simulink model "trialmk"  (R2017b)
settings: Solver=VariableStepAuto  StartTime=0.0  StopTime=10.0  RelTol=1e-3
values from neighbouring files (symbols this model uses):
  traj_freq = 1001    [basic_3link_plantraj3_emptry.m]
undefined symbols (not defined in the file or in its folder): FDab, planar
libraries: simulink x4
settings Model: Creator=USER  LastModifiedBy=USER

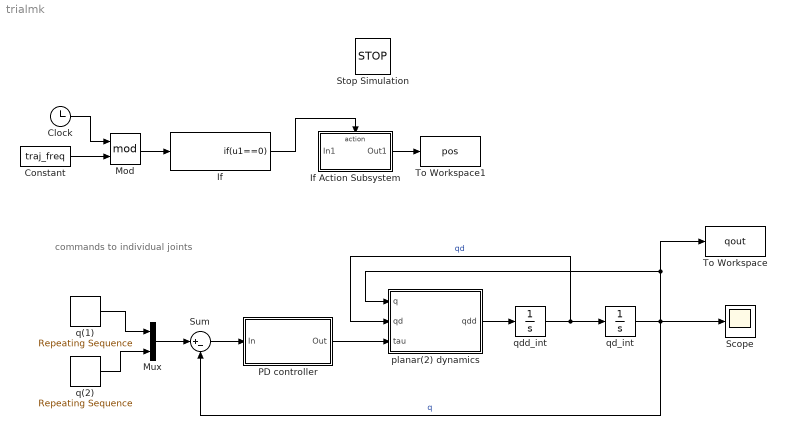
== system trialmk ==
  note: commands to
      | individual
      | joints
  Clock : Clock
  Constant : Constant  Value=traj_freq
  If : If  IfExpression=u1==0  ShowElse=off
  If Action Subsystem : Subsystem  TreatAsAtomicUnit=on
  Mod : Math  Operator=mod  SaturateOnIntegerOverflow=on
  Mux : Mux  Inputs=2
  PD controller : Subsystem
  Scope : Scope
  Stop Simulation : Stop
  Sum : Sum  Inputs=|+-
  To Workspace : ToWorkspace  VariableName=qout  SampleTime=-1
  To Workspace1 : ToWorkspace  VariableName=pos  SaveFormat=Timeseries  SampleTime=-1
  planar(2) dynamics : Subsystem
  q(1) : simulink/Sources/Repeating Sequence  rep_seq_t=[0 1 2 3 4]  rep_seq_y=pos
  q(2) : simulink/Sources/Repeating Sequence  rep_seq_t=[0 1 2 3 4]  rep_seq_y=[0 2 2 0 0]
  qd_int : Integrator
  qdd_int : Integrator
  wires:
  Mux/1 -> Sum/1
  q(2)/1 -> Mux/2
  qdd_int/1 -> qd_int/1, planar(2) dynamics/2(qd)  "qd"
  planar(2) dynamics/1(qdd) -> qdd_int/1
  Sum/1 -> PD controller/1(In)
  qd_int/1 -> Scope/1, Sum/2, planar(2) dynamics/1(q), To Workspace/1  "q"
  PD controller/1(Out) -> planar(2) dynamics/3(tau)
  Clock/1 -> Mod/1
  Mod/1 -> If/1
  Constant/1 -> Mod/2
  q(1)/1 -> Mux/1
  If Action Subsystem/1(Out1) -> To Workspace1/1
  If/1 -> If Action Subsystem/Action

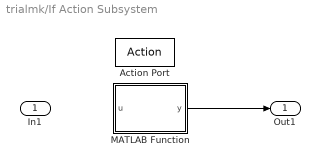
== system trialmk/If Action Subsystem ==
  In1 : Inport
  Action Port : ActionPort  ActionType=then
  MATLAB Function : MATLAB Function  TreatAsAtomicUnit=on
  Out1 : Outport
  wires:
  MATLAB Function/1(y) -> Out1/1

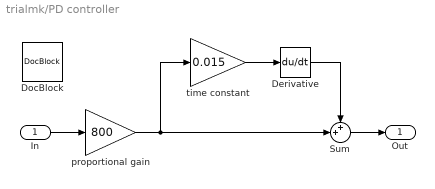
== system trialmk/PD controller ==
  In : Inport
  Derivative : Derivative
  DocBlock : simulink/Model-Wide Utilities/DocBlock  DocumentType=Text
      content=|
      | This control system is deliberately badly tuned, so that you can see the
      | dynamics in action.  Observe that the wobbling is worse, and at a lower
      | frequency, when the robot is straight than when it is bent.  Also, it is
      | mostly joint 1 that wobbles.  These are both consequences of the dynamics:
      | the robot exhibits a larger inertia about joint 1 than about joint 2,
      | meaning that a larger force is required to make joint 1 move than joint 2.
      | Furthermore, the inertia is larger when the robot is straight than when it
      | is bent.
      |
      | Once you have seen how badly this controller works, try changing the
      | gains.  For example, increasing the proportional gain (e.g. to 1500) will
      | make an obvious improvement.  Increasing the time constant will increase
      | the damping -- try increasing it to 0.05 to see what happens.  Another
      | thing you can do is make the gains different for joints 1 and 2.  For
      | example, setting the proportional gain to [1000; 100] will apply a gain of
      | 1000 to joint 1 and 100 (which is too low) to joint 2.  Now it is joint 2
      | that does most of the wobbling.
  Sum : Sum  Inputs=++|
  proportional gain : Gain  Gain=800
  time constant : Gain  Gain=0.015
  Out : Outport
  wires:
  In/1 -> proportional gain/1
  proportional gain/1 -> Sum/2, time constant/1
  time constant/1 -> Derivative/1
  Derivative/1 -> Sum/1
  Sum/1 -> Out/1

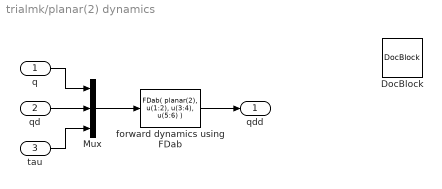
== system trialmk/planar(2) dynamics ==
  q : Inport
  qd : Inport  Port=2
  tau : Inport  Port=3
  DocBlock : simulink/Model-Wide Utilities/DocBlock  DocumentType=Text
      content=|
      | This subsystem shows the simplest method for incorporating dynamics
      | calculations into a Simulink model.  Simulink provides a "MATLAB function"
      | block, to allow Matlab functions to be incorporated into a Simulink model.
      | However, this block has only a single input and a single output.
      | Therefore, the first thing that must happen is that the three variables
      | needed for the dynamics calculation (q, qd and tau) must be combined into
      | a single vector, so that it can be fed in as the single input to the
      | Matlab function block.  If you open this block, you will find that the
      | actual function call is "FDab( planar(2), u(1:2), u(3:4), u(5:6) )".  The
      | expressions u(1:2), u(3:4) and u(5:6) extract the 2x1 vectors q, qd and
      | tau from the 6x1 input vector u, so that the call is effectively
      | "FDab( planar(2), q, qd, tau )".
      |
      | There is one more important thing to note about this block: Simulink needs
      | to be told the type and dimensions of the return value.  Now, the return
      | value (qdd) is a 2x1 vector of real numbers (because planar(2) has two
      | joint variables); so the Matlab function block's parameter "Output
      | dimensions:" has to be set to "[2 1]", the output signal type must be set
      | to "real", and the box "Collapse 2-D results to 1-D" must be un-checked.
      |
      | "planar(2)" is a call to the model-creating function "planar".  This
      | function will be called every time that FDab is called, which is several
      | times per integration step.  If planar were to create a new model every
      | time it was called, it would be an obvious piece of inefficiency.
      | However, if you look at the source code of planar (in models/planar.m),
      | you will find that it stores a copy of the last model it made, and returns
      | that copy if the argument matches.
      |
      | This style of use, in which a dynamics function (like FDab) is called
      | directly, the input vector u is explicitly split into its component parts,
      | and a model-preparation function (like planar) supplies a model at every
      | call, is the simplest way to proceed.  The only snags are: (1) you need to
      | get the numbers right, and (2) for the sake of efficiency, the
      | model-preparation function ought to use the same strategy that you see in
      | planar.  If you wanted to modify this Simulink model to use planar(3)
      | (i.e., a three-joint robot) instead of planar(2), then you would have to
      | change the function call to read
      | "FDab( planar(3), u(1:3), u(4:6), u(7:9) )", and you would have to change
      | the output dimensions to "[3 1]".  You would also have to supply a motion
      | command signal for q(3).
  Mux : Mux  Inputs=3
  forward dynamics using FDab : MATLABFcn  MATLABFcn=FDab( planar(2), u(1:2), u(3:4), u(5:6) )  OutputDimensions=[2 1]  OutputSignalType=real  Output1D=off
  qdd : Outport
  wires:
  qd/1 -> Mux/2
  q/1 -> Mux/1
  tau/1 -> Mux/3
  Mux/1 -> forward dynamics using FDab/1
  forward dynamics using FDab/1 -> qdd/1

== matlab function trialmk/If Action Subsystem/MATLAB Function ==
  data: u input; y output
function y = set_to_random(u)
y=[rand(5,1)*10]'
end
